simulink model "BESS_Harness"  (R2025b)
settings: Solver=VariableStepAuto  StartTime=0.0  StopTime=5  RelTol=1e-3
PostLoadFcn:
  | BESSParam
undefined symbols (not defined in the file): bessSystem, bessVoltage, DiscIntNeverNeededParam, gflInverter, gfmInverter, solar, Ts
libraries: eeGeneralControl x26, nesl_utility x26, ee_lib x16, simulink x12, fl_lib x10, eeTransforms x7, nesl_utility_internal x4, slpidlib x2, batteryecm_lib x2, simulink_extras x1, eePowerMeasurement x1, eePwmGenerator x1
(part 2 of 4)

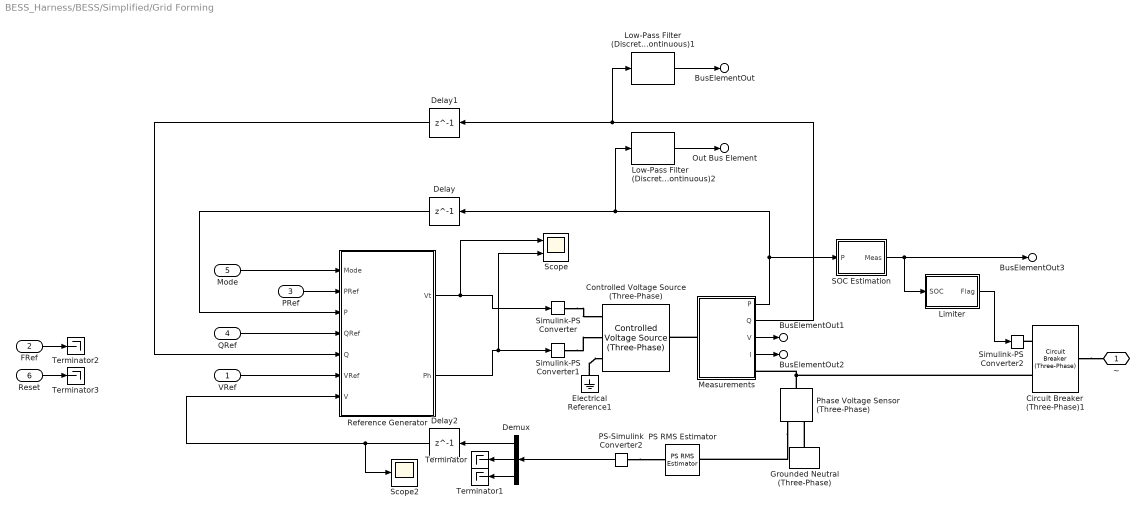
== system BESS_Harness/BESS/Simplified/Grid Forming ==
  VRef : Inport
  FRef : Inport  Port=2
  PRef : Inport  Port=3
  QRef : Inport  Port=4
  Mode : Inport  Port=5
  Reset : Inport  Port=6
  Circuit Breaker (Three-Phase)1 : ee_lib/Switches & Breakers/Circuit Breaker (Three-Phase)  R_closed=0.001 Ohm  G_open=1e-6 1/Ohm  threshold=0.5 V  breaker_behavior=ee.enum.switches.breakerBehavior.zeroCrossingDisable
      settings: InternalSimscapePortConfiguration="{\"Bottom\":[],\"Left\":[{\"id\":\"vT\",\"label\":\"vT\",\"type\":\"input\"},{\"id\":\"N1\",\"label\":\"~1\",\"type\":\"foundation.electrical.three_phase\"}],\"Right\":[{\"id\":\"N2\",\"label\":\"~2\",\"type\":\"foundation.electrical.three_phase\"}],\"Top\":[]}"
  Controlled Voltage Source (Three-Phase) : ee_lib/Sources/Controlled Voltage Source (Three-Phase)  input_option=ee.enum.inputType.singleFreqAC  FRated=frequency Hz
      settings: InternalSimscapePortConfiguration="{\"Bottom\":[],\"Left\":[{\"id\":\"Vt\",\"label\":\"Vt\",\"type\":\"input\"},{\"id\":\"ph\",\"label\":\"ph\",\"type\":\"input\"},{\"id\":\"n\",\"label\":\"n\",\"type\":\"foundation.electrical.electrical\"}],\"Right\":[{\"id\":\"N\",\"label\":\"~\",\"type\":\"foundation.electrical.three_phase\"}],\"Top\":[]}"
  Delay : Delay  DelayLength=1
  Delay1 : Delay  DelayLength=1
  Delay2 : Delay  DelayLength=1
  Demux : Demux  Outputs=3
  Electrical Reference1 : fl_lib/Electrical/Electrical Elements/Electrical Reference
  Grounded Neutral (Three-Phase) : ee_lib/Connectors & References/Grounded Neutral (Three-Phase)
  Limiter : Subsystem
  Low-Pass Filter (Discrete or Continuous)1 : eeGeneralControl/Low-Pass Filter (Discrete or Continuous)  K=1  T=0.1  B=inf  A=-inf  init_option=Inherited from block input  x0=0  Ts=-1
  Low-Pass Filter (Discrete or Continuous)2 : eeGeneralControl/Low-Pass Filter (Discrete or Continuous)  K=1  T=0.1  B=inf  A=-inf  init_option=Inherited from block input  x0=0  Ts=-1
  Measurements : Subsystem
  PS RMS Estimator : fl_lib/Physical Signals/Periodic Operators/PS RMS Estimator  f0=frequency Hz
      settings: InternalSimscapePortConfiguration="{\"Bottom\":[],\"Left\":[{\"id\":\"I\",\"label\":\"\",\"type\":\"input\"}],\"Right\":[{\"id\":\"O\",\"label\":\"\",\"type\":\"output\"}],\"Top\":[]}"
  PS-Simulink Converter2 : nesl_utility/PS-Simulink Converter  PhysicalDomain=network_engine_domain  SubClassName=ps_output  LeftPortType=input  RightPortType=output  PseudoPeriodic=off  Frequencies=[]  VectorFormat=inherit  Unit=inherit  AffineConversion=off
  Phase Voltage Sensor (Three-Phase) : ee_lib/Sensors & Transducers/Phase Voltage Sensor (Three-Phase)
  Reference Generator : Subsystem  mask{activeDroop=activeDroop, reactiveDroop=reactiveDroop, systemVoltage=Vac, systemFrequency=frequency, basePower=plantRating*1000}
      mask prompts: activeDroop "Active Droop"; reactiveDroop "Reactive Droop"; systemVoltage "AC Voltage"; systemFrequency "Frequency"; basePower "Base Power"
  SOC Estimation : Subsystem
  Scope : Scope  NumInputPorts=2
      settings: ActiveDisplayYMinimum=603.75  ActiveDisplayYMaximum=776.25000000000011
  Scope2 : Scope
  Simulink-PS Converter : nesl_utility/Simulink-PS Converter  PhysicalDomain=network_engine_domain  SubClassName=ps_input  LeftPortType=input  RightPortType=output  PseudoPeriodic=off  Frequencies=[]  NoiseDistribution=none  NoiseParameters=[]  Unit=1  AffineConversion=off  FilteringAndDerivatives=provide  SimscapeFilterOrder=1  InputFilterTimeConstant=0.001  UdotUserProvided=0
  Simulink-PS Converter1 : nesl_utility/Simulink-PS Converter  PhysicalDomain=network_engine_domain  SubClassName=ps_input  LeftPortType=input  RightPortType=output  PseudoPeriodic=off  Frequencies=[]  NoiseDistribution=none  NoiseParameters=[]  Unit=1  AffineConversion=off  FilteringAndDerivatives=provide  SimscapeFilterOrder=1  InputFilterTimeConstant=0.001  UdotUserProvided=0
  Simulink-PS Converter2 : nesl_utility/Simulink-PS Converter  PhysicalDomain=network_engine_domain  SubClassName=ps_input  LeftPortType=input  RightPortType=output  PseudoPeriodic=off  Frequencies=[]  NoiseDistribution=none  NoiseParameters=[]  Unit=1  AffineConversion=off  FilteringAndDerivatives=provide  SimscapeFilterOrder=1  InputFilterTimeConstant=0.001  UdotUserProvided=0
  Terminator{,1..3} (4 alike) : Terminator
  ~ : PMIOPort  Side=Right
  Out Bus Element : Outport  PortName=Meas  Element=activePower
  BusElementOut : Outport  PortName=Meas  Element=reactivePower
  BusElementOut1 : Outport  PortName=Meas  Element=voltage
  BusElementOut2 : Outport  PortName=Meas  Element=current
  BusElementOut3 : Outport  PortName=Meas  Element=SOC
  wires:
  Limiter/1(Flag) -> Simulink-PS Converter2/1
  PRef/1 -> Reference Generator/2(PRef)
  Low-Pass Filter (Discrete or Continuous)2/1 -> Out Bus Element/1
  Low-Pass Filter (Discrete or Continuous)1/1 -> BusElementOut/1
  Mode/1 -> Reference Generator/1(Mode)
  Delay1/1 -> Reference Generator/5(Q)
  FRef/1 -> Terminator2/1
  Reference Generator/1(Vt) -> Scope/1, Simulink-PS Converter/1
  VRef/1 -> Reference Generator/6(VRef)
  QRef/1 -> Reference Generator/4(QRef)
  Demux/1 -> Delay2/1
  Delay/1 -> Reference Generator/3(P)
  PS-Simulink Converter2/1 -> Demux/1
  Reference Generator/2(Ph) -> Scope/2, Simulink-PS Converter1/1
  Demux/2 -> Terminator/1
  Delay2/1 -> Reference Generator/7(V), Scope2/1
  Reset/1 -> Terminator3/1
  Demux/3 -> Terminator1/1
  Measurements/1(P) -> SOC Estimation/1(P), Low-Pass Filter (Discrete or Continuous)2/1, Delay/1
  Measurements/2(Q) -> Low-Pass Filter (Discrete or Continuous)1/1, Delay1/1
  Measurements/3(V) -> BusElementOut1/1
  Measurements/4(I) -> BusElementOut2/1
  SOC Estimation/1(Meas) -> Limiter/1(SOC), BusElementOut3/1
  connections:
  Circuit Breaker (Three-Phase)1/LConn1 -- Simulink-PS Converter2/RConn1
  Circuit Breaker (Three-Phase)1/RConn1 -- ~/RConn1
  PS-Simulink Converter2/LConn1 -- PS RMS Estimator/RConn1
  Measurements/LConn1 -- Controlled Voltage Source (Three-Phase)/RConn1
  Simulink-PS Converter1/RConn1 -- Controlled Voltage Source (Three-Phase)/LConn2
  Electrical Reference1/LConn1 -- Controlled Voltage Source (Three-Phase)/LConn3
  Circuit Breaker (Three-Phase)1/LConn2 -- Phase Voltage Sensor (Three-Phase)/LConn1 -- Measurements/RConn1
  Phase Voltage Sensor (Three-Phase)/RConn1 -- PS RMS Estimator/LConn1
  Simulink-PS Converter/RConn1 -- Controlled Voltage Source (Three-Phase)/LConn1
  Grounded Neutral (Three-Phase)/LConn1 -- Phase Voltage Sensor (Three-Phase)/RConn2

== system BESS_Harness/BESS/Detailed/BESS Controller/Grid Following ==
  VRef : Inport
  FRef : Inport  Port=2
  PRef : Inport  Port=3
  QRef : Inport  Port=4
  Mode : Inport  Port=5
  Reset : Inport  Port=6
  In Bus Element3 : Inport  Port=7  PortName=VIBus  Element=Vd
  BusElementIn : Inport  Port=7  PortName=VIBus  Element=Vd
  In Bus Element2 : Inport  Port=7  PortName=VIBus  Element=Vq
  In Bus Element7 : Inport  Port=7  PortName=VIBus  Element=Theta
  BusElementIn1 : Inport  Port=7  PortName=VIBus  Element=Freq
  BusElementIn3 : Inport  Port=7  PortName=VIBus  Element=Id
  BusElementIn4 : Inport  Port=7  PortName=VIBus  Element=Iq
  Constant : Constant  Value=10
  Current_controller : Subsystem
  Inverse Park Transform1 : eeTransforms/Inverse Park Transform  AxisAlignment=Q-axis  PowerInvariant=off
  Reference Current : Subsystem
  Sum2 : Sum  Inputs=|+-
  Terminator : Terminator
  Terminator1 : Terminator
  Unit Delay : UnitDelay  SampleTime=Td
  Unit Delay1 : UnitDelay  SampleTime=Td
  Unit Delay2 : UnitDelay  SampleTime=Ts
  mabc : Outport
  wires:
  QRef/1 -> Reference Current/6(QRef)
  PRef/1 -> Reference Current/5(PRef)
  BusElementIn4/1 -> Current_controller/4(iq)
  BusElementIn3/1 -> Current_controller/2(ipvd)
  BusElementIn1/1 -> Unit Delay1/1
  BusElementIn/1 -> Unit Delay/1
  Unit Delay/1 -> Reference Current/2(V-mag)
  Unit Delay1/1 -> Sum2/2
  Reference Current/1(id_ref) -> Current_controller/1(id-ref)
  Reference Current/2(iq_ref) -> Current_controller/3(iqref)
  Sum2/1 -> Reference Current/3(del f)
  VRef/1 -> Reference Current/1(V_ref)
  FRef/1 -> Sum2/1
  In Bus Element7/1 -> Inverse Park Transform1/2
  In Bus Element3/1 -> Current_controller/5(Vd)
  Current_controller/1(mdq0) -> Inverse Park Transform1/1
  Unit Delay2/1 -> mabc/1
  Inverse Park Transform1/1 -> Unit Delay2/1
  In Bus Element2/1 -> Current_controller/6(Vq)
  Mode/1 -> Terminator/1
  Reset/1 -> Terminator1/1
  Constant/1 -> Reference Current/4(LVRT_iq)

== system BESS_Harness/BESS/Detailed/BESS Controller/Grid Forming ==
  VRef : Inport
  FRef : Inport  Port=2
  PRef : Inport  Port=3
  QRef : Inport  Port=4
  Mode : Inport  Port=5
  Reset : Inport  Port=6
  Bus Element In : Inport  Port=7  PortName=VIBus  Element=Vabc
  BusElementIn : Inport  Port=7  PortName=VIBus  Element=Iabc
  Current Limiting : Subsystem
  Grid Voltage Reactive Power Support : Subsystem
  Measurement : Subsystem
      mask Display: image('meas2_1_7_7_2.png');
  Power Control : Subsystem
  Subsystem2 : Subsystem
      settings: PortSchema="{\"entries\":[{\"content\":{\"sides\":[{\"content\":{\"connectorIds\":[\"Out1\"]},\"type\":\"ConnectorPlacement.EquallySpacedRectSide\",\"uuid\":\"7526c1f7-0aba-4355-8bbd-47d168879ecb\"},{\"content\":{\"connectorIds\":[\"In1\",\"In2\"],\"side\":\"RIGHT\"},\"type\":\"ConnectorPlacement.EquallySpacedRectSide\",\"uuid\":\"1dda9693-ec76-4df0-8ad4-aaa83d2574b3\"},{\"content\":{\"side\":\"TOP\"},\"type\":\"ConnectorPlacement.EquallySpacedRectSide\",\"uuid\":\"71ea411b-eb5f-4279-ae23-08ebb3ff1ed6\"}]},\"type\":\"ConnectorPlacement.EquallySpacedConnector\",\"uuid\":\"19864e0c-0998-460d-9705-13c69283d4ec\"}],\"packageUris\":[\"http://schema.mathworks.com/mf0/Connector/R2020b\"],\"version\":\"1.0\"}"
  Terminator : Terminator
  Terminator1 : Terminator
  Terminator2 : Terminator
  VoltageCurrentControl : Subsystem
      settings: PortSchema="{\"entries\":[{\"content\":{\"sides\":[{\"content\":{\"connectorIds\":[\"In1\",\"In2\",\"In3\"]},\"type\":\"ConnectorPlacement.EquallySpacedRectSide\",\"uuid\":\"0bf15a12-7bc0-47e4-89bd-435769673763\"},{\"content\":{\"connectorIds\":[\"Out1\"],\"side\":\"RIGHT\"},\"type\":\"ConnectorPlacement.EquallySpacedRectSide\",\"uuid\":\"44a15d74-8878-4ec6-abe4-be0b1b609519\"},{\"content\":{\"connectorIds\":[\"In4\"],\"side\":\"TOP\"},\"type\":\"ConnectorPlacement.EquallySpacedRectSide\",\"uuid\":\"7a96781e-5638-4b2a-8101-d5785aae9f0f\"}]},\"type\":\"ConnectorPlacement.EquallySpacedConnector\",\"uuid\":\"4b3373ad-cf20-4175-894e-3bd1604dd0ce\"}],\"packageUris\":[\"http://schema.mathworks.com/mf0/Connector/R2020b\"],\"version\":\"1.0\"}"
  mabc : Outport
  wires:
  Reset/1 -> Subsystem2/2(Reset), VoltageCurrentControl/3(Reset)
  Mode/1 -> Power Control/6(CntrlFlag)
  VRef/1 -> Power Control/4(Vref)
  FRef/1 -> Power Control/5(Fref)
  Measurement/4(fmeas) -> Terminator2/1
  Grid Voltage Reactive Power Support/2(Qref) -> Power Control/3(Qref)
  Grid Voltage Reactive Power Support/1(Pref) -> Power Control/2(Pref)
  PRef/1 -> Grid Voltage Reactive Power Support/2(PrefInput)
  QRef/1 -> Grid Voltage Reactive Power Support/3(QrefInput)
  Current Limiting/1(currentLimiting) -> VoltageCurrentControl/1(currentLimiting)
  Power Control/2(activeControl) -> VoltageCurrentControl/2(activeControl)
  Power Control/1(reactiveControl) -> Current Limiting/2(reactiveControl)
  Power Control/3(angle) -> Measurement/3(Angle)
  Measurement/1(measure) -> Grid Voltage Reactive Power Support/1(measure), Power Control/1(measure), VoltageCurrentControl/4(measure), Current Limiting/1(measure)
  Measurement/3(Qmeas) -> Terminator1/1
  Measurement/2(Pmeas) -> Terminator/1
  BusElementIn/1 -> Measurement/2(Igabc)
  Bus Element In/1 -> Measurement/1(Vgabcc)
  VoltageCurrentControl/1(mabc) -> Subsystem2/1(In)
  Subsystem2/1(mabc) -> mabc/1

== system BESS_Harness/BESS/Detailed/BESS Plant/Converter ==
  mabc : Inport
  Average : Subsystem  VariantControl=Average
  Switching : Subsystem  VariantControl=Switching
  + : PMIOPort  Side=Left
  - : PMIOPort  Port=2  Side=Left
  ~ : PMIOPort  Port=3  Side=Right

== system BESS_Harness/BESS/Detailed/Filter & Measurements/PLL & Measurements ==
  V : Inport
  I : Inport  Port=2
  Measurement1 : Subsystem
  Measurement2 : Subsystem
  Subsystem : Subsystem
  Out Bus Element : Outport  PortName=VIbus  Element=Vq
  Out Bus Element1 : Outport  PortName=VIbus  Element=Vd
  Out Bus Element2 : Outport  PortName=VIbus  Element=Freq
  Out Bus Element3 : Outport  PortName=VIbus  Element=Theta
  Out Bus Element4 : Outport  PortName=VIbus  Element=Vmag
  Out Bus Element5 : Outport  PortName=VIbus  Element=Iq
  Out Bus Element6 : Outport  PortName=VIbus  Element=Id
  Out Bus Element7 : Outport  PortName=VIbus  Element=Iabc
  Out Bus Element8 : Outport  PortName=VIbus  Element=Vabc
  wires:
  Subsystem/6(Id1) -> Out Bus Element6/1
  Subsystem/7(Iq1) -> Out Bus Element5/1
  Measurement1/1(Vg) -> Subsystem/2(Iabc), Out Bus Element7/1
  I/1 -> Measurement1/1(u)
  Subsystem/1(mag) -> Out Bus Element4/1
  Measurement2/1(Vg) -> Subsystem/1(Vabc), Out Bus Element8/1
  Subsystem/4(Vd) -> Out Bus Element1/1
  Subsystem/3(angle) -> Out Bus Element3/1
  Subsystem/5(Vq) -> Out Bus Element/1
  Subsystem/2(freq) -> Out Bus Element2/1
  V/1 -> Measurement2/1(u)

== system BESS_Harness/BESS/Simplified/Grid Following/Measurements ==
  Current and Voltage Sensor (Three-Phase)1 : ee_lib/Sensors & Transducers/Current and Voltage Sensor (Three-Phase)  vMeasurementType=ee.enum.vmeasurement.lg  outputUnit=ee.enum.unit.pu  SRated=plantRating*1000 A*V  VRated=Vac V  I_specify=off  I_priority=None  I=[0, 0, 0] A  I_nominal_specify=off  I_nominal_value=1  I_nominal_unit=A  V_specify=off  V_priority=None  V=[0, 0, 0] V  V_nominal_specify=off  V_nominal_value=1  V_nominal_unit=V
      settings: InternalSimscapePortConfiguration="{\"Bottom\":[],\"Left\":[{\"id\":\"N1\",\"label\":\"~1\",\"type\":\"foundation.electrical.three_phase\"}],\"Right\":[{\"id\":\"V_output\",\"label\":\"V\",\"type\":\"output\"},{\"id\":\"I_output\",\"label\":\"I\",\"type\":\"output\"},{\"id\":\"N2\",\"label\":\"~2\",\"type\":\"foundation.electrical.three_phase\"}],\"Top\":[]}"
  Gain1 : Gain  Gain=1/(plantRating*1000)
  Gain2 : Gain  Gain=1/(plantRating*1000)
  Low-Pass Filter (Discrete or Continuous)1 : eeGeneralControl/Low-Pass Filter (Discrete or Continuous)  K=1  T=0.1  B=inf  A=-inf  init_option=Inherited from block input  x0=0  Ts=-1
  Low-Pass Filter (Discrete or Continuous)2 : eeGeneralControl/Low-Pass Filter (Discrete or Continuous)  K=1  T=0.1  B=inf  A=-inf  init_option=Inherited from block input  x0=0  Ts=-1
  PS-Simulink Converter{,1..3} (4 alike) : nesl_utility/PS-Simulink Converter  PhysicalDomain=network_engine_domain  SubClassName=ps_output  LeftPortType=input  RightPortType=output  PseudoPeriodic=off  Frequencies=[]  VectorFormat=inherit  Unit=inherit  AffineConversion=off
  Power Sensor (Three-Phase) : ee_lib/Sensors & Transducers/Power Sensor (Three-Phase)  load_type=ee.enum.passive.type_balanced.balanced  f0=60 Hz
      settings: InternalSimscapePortConfiguration="{\"Bottom\":[],\"Left\":[{\"id\":\"N1\",\"label\":\"~1\",\"type\":\"foundation.electrical.three_phase\"}],\"Right\":[{\"id\":\"N2\",\"label\":\"~2\",\"type\":\"foundation.electrical.three_phase\"}],\"Top\":[{\"id\":\"Pm\",\"label\":\"P\",\"type\":\"output\"},{\"id\":\"Qm\",\"label\":\"Q\",\"type\":\"output\"}]}"
  In : PMIOPort  Side=Left
  ~ : PMIOPort  Port=2  Side=Right
  P : Outport
  Q : Outport  Port=2
  V : Outport  Port=3
  I : Outport  Port=4
  wires:
  Gain2/1 -> Q/1
  Gain1/1 -> P/1
  PS-Simulink Converter3/1 -> I/1
  PS-Simulink Converter2/1 -> V/1
  Low-Pass Filter (Discrete or Continuous)2/1 -> Gain2/1
  Low-Pass Filter (Discrete or Continuous)1/1 -> Gain1/1
  PS-Simulink Converter1/1 -> Low-Pass Filter (Discrete or Continuous)2/1
  PS-Simulink Converter/1 -> Low-Pass Filter (Discrete or Continuous)1/1
  connections:
  Current and Voltage Sensor (Three-Phase)1/RConn2 -- PS-Simulink Converter3/LConn1
  Current and Voltage Sensor (Three-Phase)1/LConn1 -- Power Sensor (Three-Phase)/RConn1
  PS-Simulink Converter1/LConn1 -- Power Sensor (Three-Phase)/LConn3
  Current and Voltage Sensor (Three-Phase)1/RConn3 -- ~/RConn1
  In/RConn1 -- Power Sensor (Three-Phase)/LConn1
  PS-Simulink Converter/LConn1 -- Power Sensor (Three-Phase)/LConn2
  Current and Voltage Sensor (Three-Phase)1/RConn1 -- PS-Simulink Converter2/LConn1

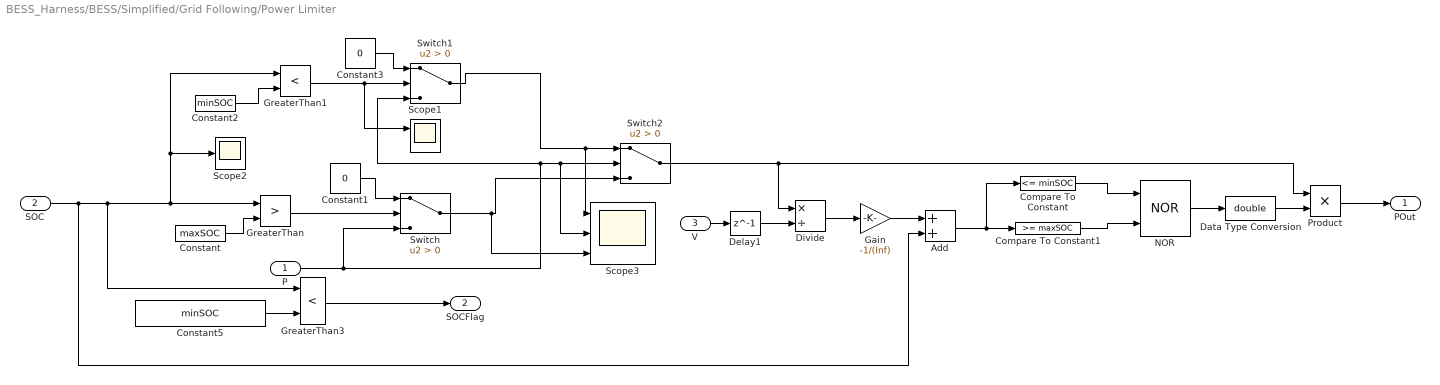
== system BESS_Harness/BESS/Simplified/Grid Following/Power Limiter ==
  P : Inport
  SOC : Inport  Port=2
  V : Inport  Port=3
  Add : Sum
  Compare To Constant : simulink/Logic and Bit Operations/Compare To Constant  relop=<=  const=minSOC  OutDataTypeStr=boolean
  Compare To Constant1 : simulink/Logic and Bit Operations/Compare To Constant  relop=>=  const=maxSOC  OutDataTypeStr=boolean
  Constant : Constant  Value=maxSOC
  Constant1 : Constant  Value=0
  Constant2 : Constant  Value=minSOC
  Constant3 : Constant  Value=0
  Constant5 : Constant  Value=minSOC
  Data Type Conversion : DataTypeConversion  OutDataTypeStr=double  SaturateOnIntegerOverflow=off  RndMeth=Floor
  Delay1 : Delay  DelayLength=1
  Divide : Product  Inputs=*/
  Gain : Gain  Gain=-1/(Inf)
  GreaterThan : RelationalOperator  Operator=>  OutDataTypeStr=boolean  RndMeth=Simplest  InputSameDT=off
  GreaterThan1 : RelationalOperator  Operator=<  OutDataTypeStr=boolean  RndMeth=Simplest  InputSameDT=off
  GreaterThan3 : RelationalOperator  Operator=<  OutDataTypeStr=boolean  RndMeth=Simplest  InputSameDT=off
  NOR : Logic  Operator=NOR  IconShape=distinctive  AllPortsSameDT=off  OutDataTypeStr=boolean
  Product : Product
  Scope1 : Scope  NumInputPorts=2
  Scope2 : Scope
  Scope3 : Scope  NumInputPorts=3
  Switch : Switch  Criteria=u2 > Threshold  SaturateOnIntegerOverflow=off  InputSameDT=off
  Switch1 : Switch  Criteria=u2 > Threshold  SaturateOnIntegerOverflow=off  InputSameDT=off
  Switch2 : Switch  Criteria=u2 > Threshold  SaturateOnIntegerOverflow=off  InputSameDT=off
  POut : Outport
  SOCFlag : Outport  Port=2
  wires:
  Product/1 -> POut/1
  Gain/1 -> Add/1
  Data Type Conversion/1 -> Product/2
  NOR/1 -> Data Type Conversion/1
  Compare To Constant1/1 -> NOR/2
  Compare To Constant/1 -> NOR/1
  Add/1 -> Compare To Constant1/1, Compare To Constant/1
  Switch2/1 -> Product/1, Divide/1
  Switch/1 -> Switch2/3, Scope3/3
  SOC/1 -> GreaterThan/1, GreaterThan1/1, Scope2/1, GreaterThan3/1, Add/2
  Divide/1 -> Gain/1
  Delay1/1 -> Divide/2
  V/1 -> Delay1/1
  GreaterThan3/1 -> SOCFlag/1
  Constant5/1 -> GreaterThan3/2
  Constant/1 -> GreaterThan/2
  GreaterThan/1 -> Switch/2
  Constant1/1 -> Switch/1
  Constant2/1 -> GreaterThan1/2
  GreaterThan1/1 -> Switch1/2, Scope1/1
  Constant3/1 -> Switch1/1
  Switch1/1 -> Switch2/1, Scope3/1
  P/1 -> Switch/3, Switch1/3, Switch2/2, Scope3/2

== system BESS_Harness/BESS/Simplified/Grid Following/SOC Estimation ==
  I : Inport
  Constant : Constant  Value=0.95
  Gain : Gain  Gain=-1/(100000)
  Integrator (Discrete or Continuous) : eeGeneralControl/Integrator (Discrete or Continuous)  LabelModeActiveChoice=Discrete  IntegratorMethod=Integration: Forward Euler  ExternalReset=level  LimitType=Anti-windup  B=inf  A=-inf  Ts=-1
  SOC : Outport
  wires:
  Integrator (Discrete or Continuous)/1 -> SOC/1
  Gain/1 -> Integrator (Discrete or Continuous)/1
  I/1 -> Gain/1
  Constant/1 -> Integrator (Discrete or Continuous)/3

== system BESS_Harness/BESS/Simplified/Grid Forming/Limiter ==
  SOC : Inport
  Compare To Constant : simulink/Logic and Bit Operations/Compare To Constant  relop=<=  const=minSOC  OutDataTypeStr=boolean
  Compare To Constant1 : simulink/Logic and Bit Operations/Compare To Constant  relop=>=  const=maxSOC  OutDataTypeStr=boolean
  Data Type Conversion : DataTypeConversion  OutDataTypeStr=double  SaturateOnIntegerOverflow=off  RndMeth=Floor
  Delay : Delay  DelayLength=1  InputProcessing=Columns as channels (frame based)
  OR : Logic  Operator=OR  AllPortsSameDT=off  OutDataTypeStr=boolean
  Flag : Outport
  wires:
  Delay/1 -> Flag/1
  Data Type Conversion/1 -> Delay/1
  OR/1 -> Data Type Conversion/1
  Compare To Constant1/1 -> OR/2
  Compare To Constant/1 -> OR/1
  SOC/1 -> Compare To Constant1/1, Compare To Constant/1

== system BESS_Harness/BESS/Simplified/Grid Forming/Measurements ==
  Current and Voltage Sensor (Three-Phase)5 : ee_lib/Sensors & Transducers/Current and Voltage Sensor (Three-Phase)  vMeasurementType=ee.enum.vmeasurement.lg  outputUnit=ee.enum.unit.pu  SRated=plantRating*1000 A*V  VRated=Vac V  I_specify=off  I_priority=None  I=[0, 0, 0] A  I_nominal_specify=off  I_nominal_value=1  I_nominal_unit=A  V_specify=off  V_priority=None  V=[0, 0, 0] V  V_nominal_specify=off  V_nominal_value=1  V_nominal_unit=V
      settings: InternalSimscapePortConfiguration="{\"Bottom\":[],\"Left\":[{\"id\":\"N1\",\"label\":\"~1\",\"type\":\"foundation.electrical.three_phase\"}],\"Right\":[{\"id\":\"V_output\",\"label\":\"V\",\"type\":\"output\"},{\"id\":\"I_output\",\"label\":\"I\",\"type\":\"output\"},{\"id\":\"N2\",\"label\":\"~2\",\"type\":\"foundation.electrical.three_phase\"}],\"Top\":[]}"
  Gain1 : Gain  Gain=1/(plantRating*1000)
  Gain2 : Gain  Gain=1/(plantRating*1000)
  PS-Simulink Converter{,1..3} (4 alike) : nesl_utility/PS-Simulink Converter  PhysicalDomain=network_engine_domain  SubClassName=ps_output  LeftPortType=input  RightPortType=output  PseudoPeriodic=off  Frequencies=[]  VectorFormat=inherit  Unit=inherit  AffineConversion=off
  Power Sensor (Three-Phase) : ee_lib/Sensors & Transducers/Power Sensor (Three-Phase)  load_type=ee.enum.passive.type_balanced.balanced  f0=60 Hz
      settings: InternalSimscapePortConfiguration="{\"Bottom\":[],\"Left\":[{\"id\":\"N1\",\"label\":\"~1\",\"type\":\"foundation.electrical.three_phase\"}],\"Right\":[{\"id\":\"N2\",\"label\":\"~2\",\"type\":\"foundation.electrical.three_phase\"}],\"Top\":[{\"id\":\"Pm\",\"label\":\"P\",\"type\":\"output\"},{\"id\":\"Qm\",\"label\":\"Q\",\"type\":\"output\"}]}"
  In : PMIOPort  Side=Left
  ~ : PMIOPort  Port=2  Side=Right
  P : Outport
  Q : Outport  Port=2
  V : Outport  Port=3
  I : Outport  Port=4
  wires:
  PS-Simulink Converter1/1 -> Gain2/1
  PS-Simulink Converter/1 -> Gain1/1
  PS-Simulink Converter2/1 -> V/1
  PS-Simulink Converter3/1 -> I/1
  Gain1/1 -> P/1
  Gain2/1 -> Q/1
  connections:
  PS-Simulink Converter2/LConn1 -- Current and Voltage Sensor (Three-Phase)5/RConn1
  PS-Simulink Converter/LConn1 -- Power Sensor (Three-Phase)/LConn2
  In/RConn1 -- Power Sensor (Three-Phase)/LConn1
  ~/RConn1 -- Current and Voltage Sensor (Three-Phase)5/RConn3
  PS-Simulink Converter1/LConn1 -- Power Sensor (Three-Phase)/LConn3
  Power Sensor (Three-Phase)/RConn1 -- Current and Voltage Sensor (Three-Phase)5/LConn1
  PS-Simulink Converter3/LConn1 -- Current and Voltage Sensor (Three-Phase)5/RConn2

== system BESS_Harness/BESS/Simplified/Grid Forming/Reference Generator ==
  Mode : Inport
  PRef : Inport  Port=2
  P : Inport  Port=3
  QRef : Inport  Port=4
  Q : Inport  Port=5
  VRef : Inport  Port=6
  V : Inport  Port=7
  Gain : Gain  Gain=efficiency/100
  Gain2 : Gain  Gain=sqrt(3)/Vac
  If : If
  If Action Subsystem : Subsystem  TreatAsAtomicUnit=on
  If Action Subsystem1 : Subsystem  TreatAsAtomicUnit=on
  Merge : Merge
  Merge1 : Merge
  Vt : Outport
  Ph : Outport  Port=2
  wires:
  Gain/1 -> If Action Subsystem/1(PRef)
  Mode/1 -> If/1
  If/1 -> If Action Subsystem/Action
  PRef/1 -> Gain/1, If Action Subsystem1/1(PRef)
  QRef/1 -> If Action Subsystem/3(QRef)
  VRef/1 -> If Action Subsystem1/3(VRef)
  V/1 -> Gain2/1
  If/2 -> If Action Subsystem1/Action
  If Action Subsystem/1(Vt) -> Merge/1
  If Action Subsystem1/1(Vt) -> Merge/2
  If Action Subsystem/2(Ph) -> Merge1/1
  If Action Subsystem1/2(Ph) -> Merge1/2
  Merge1/1 -> Ph/1
  P/1 -> If Action Subsystem/2(P), If Action Subsystem1/2(P)
  Q/1 -> If Action Subsystem/4(Q)
  Gain2/1 -> If Action Subsystem1/4(V)
  Merge/1 -> Vt/1

== system BESS_Harness/BESS/Simplified/Grid Forming/SOC Estimation ==
  P : Inport
  Constant : Constant  Value=Vdc
  Constant1 : Constant  Value=initialSOC
  Constant2 : Constant  Value=capacity
  Constant3 : Constant  Value=Inf
  Divide : Product  Inputs=*/
  Divide1 : Product  Inputs=*/
  Gain : Gain  Gain=-plantRating*1000
  Integrator (Discrete or Continuous) : eeGeneralControl/Integrator (Discrete or Continuous)  LabelModeActiveChoice=Discrete  IntegratorMethod=Integration: Forward Euler  ExternalReset=level  LimitType=Anti-windup  B=inf  A=-inf  Ts=-1
  String Compare : StringCompare
  String Constant : StringConstant  String=capacityType
  String Constant1 : StringConstant  String="\"Fixed\""
  Switch : Switch  Criteria=u2 > Threshold  SaturateOnIntegerOverflow=off  InputSameDT=off
  Meas : Outport
  wires:
  Gain/1 -> Divide/1
  P/1 -> Gain/1
  Constant/1 -> Divide/2
  Divide/1 -> Divide1/1
  Constant1/1 -> Integrator (Discrete or Continuous)/3
  Integrator (Discrete or Continuous)/1 -> Meas/1
  String Constant/1 -> String Compare/1
  String Constant1/1 -> String Compare/2
  String Compare/1 -> Switch/2
  Switch/1 -> Divide1/2
  Divide1/1 -> Integrator (Discrete or Continuous)/1
  Constant2/1 -> Switch/1
  Constant3/1 -> Switch/3

== system BESS_Harness/BESS/Detailed/BESS Controller/Grid Following/Current_controller ==
  id-ref : Inport
  ipvd : Inport  Port=2
  iqref : Inport  Port=3
  iq : Inport  Port=4
  Vd : Inport  Port=5
  Vq : Inport  Port=6
  Constant4 : Constant  Value=0
  Gain1 : Gain  Gain=2*1*pi*frequency*L/zbase
  Gain2 : Gain  Gain=2*1*pi*frequency*L/zbase
  Mux1 : Mux  Inputs=3
  PID Controller : slpidlib/PID Controller  Controller=PID  Form=Parallel  TimeDomain=Discrete-time  UseExternalTs=off  SampleTime=-1  IntegratorMethod=Forward Euler  FilterMethod=Forward Euler  ControllerParametersSource=internal  P=Kpic  I=Kiic  UseKiTs=off  D=Kd  UseExternalDerivativeSource=off  N=100  UseFilter=on  TunerSelectOption=Transfer Function Based (PID Tuner App)  InitialConditionSource=internal  InitialConditionForIntegrator=0  InitialConditionForFilter=0  DifferentiatorICPrevScaledInput=0  ExternalReset=none  TrackingMode=off  Kt=1  LimitOutput=off  SatLimitsSource=internal  UpperSaturationLimit=inf  LowerSaturationLimit=-inf  LinearizeAsGain=on  AntiWindupMode=none  Kb=1  LimitIntegrator=off  UpperIntegratorSaturationLimit=inf  LowerIntegratorSaturationLimit=-inf  POutMin=[]  POutMax=[]  IOutMin=[]  IOutMax=[]  DOutMin=[]  DOutMax=[]  NOutMin=[]  NOutMax=[]  SumOutMin=[]  SumOutMax=[]  SaturationOutMin=[]  SaturationOutMax=[]  PParamMin=[]  PParamMax=[]  IParamMin=[]  IParamMax=[]  DParamMin=[]  DParamMax=[]  NParamMin=[]  NParamMax=[]  KbParamMin=[]  KbParamMax=[]  KtParamMin=[]  KtParamMax=[]  KbOutMin=[]  KbOutMax=[]  KtOutMin=[]  KtOutMax=[]  IntegratorOutMin=[]  IntegratorOutMax=[]  FilterOutMin=[]  FilterOutMax=[]  SumI1OutMin=[]  SumI1OutMax=[]  SumI2OutMin=[]  SumI2OutMax=[]  SumI3OutMin=[]  SumI3OutMax=[]  SumI4OutMin=[]  SumI4OutMax=[]  SumDOutMin=[]  SumDOutMax=[]  DifferentiatorOutMin=[]  DifferentiatorOutMax=[]  FilterDiffOutCoefMin=[]  FilterDiffOutCoefMax=[]  ReciprocalOutMin=[]  ReciprocalOutMax=[]  SumDenOutMin=[]  SumDenOutMax=[]  SumNumOutMin=[]  SumNumOutMax=[]  DivideOutMin=[]  DivideOutMax=[]  UdiffTsProdOutMin=[]  UdiffTsProdOutMax=[]  NTsProdOutMin=[]  NTsProdOutMax=[]  UintegralTsProdOutMin=[]  UintegralTsProdOutMax=[]  UngainTsProdOutMin=[]  UngainTsProdOutMax=[]  ClampingZeroOutDataTypeStr=Inherit: Inherit via back propagation  ClampingZeroOutMin=[]  ClampingZeroOutMax=[]  FilterDenConstantOutDataTypeStr=Inherit: Inherit via back propagation  FilterDenConstantOutMin=[]  FilterDenConstantOutMax=[]  PCopyOutDataTypeStr=Inherit: Inherit via back propagation  PCopyOutMin=[]  PCopyOutMax=[]  NCopyOutDataTypeStr=Inherit: Inherit via back propagation  NCopyOutMin=[]  NCopyOutMax=[]  IntegratorContinuousStateAttributes=''  IntegratorStateMustResolveToSignalObject=off  IntegratorRTWStateStorageClass=Auto  FilterContinuousStateAttributes=''  FilterStateMustResolveToSignalObject=off  FilterRTWStateStorageClass=Auto  ParallelPVariant=InternalParameters  IdealPVariant=Disabled  IVariant=InternalParameters  DVariant=InternalParameters  IntegratorVariant=Discrete  SatVariant=Disabled  AWVariant=Passthrough  PCopyVariant=Disabled  TRVariant=Disabled  FdbkBlocksVariant=Forward  IdealPFdbkVariant=Disabled  SatFdbkVariant=Disabled  DerivativeFilterVariant=ForwardEulerFilter  NVariant=InternalParameters  NCopyVariant=Disabled  FilterICVariant=InternalICsFilter  IntegratorICVariant=InternalICs  ExternalResetVariant=Disabled  TRSumVariant=Passthrough  SumFdbkVariant=Disabled  SumVariant=Sum_PID  TsampFilterVariant=InternalTs  TsampNgainVariant=Passthrough  TsampIntegralVariant=Disabled_SignalSpec  ExternalSaturationOutDataTypeStr=Inherit: Same as second input  DerivativeSourceVariant=ErrorSignal  PreIntVariant=InternalPreInt
  PID Controller1 : slpidlib/PID Controller  Controller=PID  Form=Parallel  TimeDomain=Discrete-time  UseExternalTs=off  SampleTime=-1  IntegratorMethod=Forward Euler  FilterMethod=Forward Euler  ControllerParametersSource=internal  P=Kpic  I=Kiic  UseKiTs=off  D=Kd  UseExternalDerivativeSource=off  N=100  UseFilter=on  TunerSelectOption=Transfer Function Based (PID Tuner App)  InitialConditionSource=internal  InitialConditionForIntegrator=0  InitialConditionForFilter=0  DifferentiatorICPrevScaledInput=0  ExternalReset=none  TrackingMode=off  Kt=1  LimitOutput=off  SatLimitsSource=internal  UpperSaturationLimit=inf  LowerSaturationLimit=-inf  LinearizeAsGain=on  AntiWindupMode=none  Kb=1  LimitIntegrator=off  UpperIntegratorSaturationLimit=inf  LowerIntegratorSaturationLimit=-inf  POutMin=[]  POutMax=[]  IOutMin=[]  IOutMax=[]  DOutMin=[]  DOutMax=[]  NOutMin=[]  NOutMax=[]  SumOutMin=[]  SumOutMax=[]  SaturationOutMin=[]  SaturationOutMax=[]  PParamMin=[]  PParamMax=[]  IParamMin=[]  IParamMax=[]  DParamMin=[]  DParamMax=[]  NParamMin=[]  NParamMax=[]  KbParamMin=[]  KbParamMax=[]  KtParamMin=[]  KtParamMax=[]  KbOutMin=[]  KbOutMax=[]  KtOutMin=[]  KtOutMax=[]  IntegratorOutMin=[]  IntegratorOutMax=[]  FilterOutMin=[]  FilterOutMax=[]  SumI1OutMin=[]  SumI1OutMax=[]  SumI2OutMin=[]  SumI2OutMax=[]  SumI3OutMin=[]  SumI3OutMax=[]  SumI4OutMin=[]  SumI4OutMax=[]  SumDOutMin=[]  SumDOutMax=[]  DifferentiatorOutMin=[]  DifferentiatorOutMax=[]  FilterDiffOutCoefMin=[]  FilterDiffOutCoefMax=[]  ReciprocalOutMin=[]  ReciprocalOutMax=[]  SumDenOutMin=[]  SumDenOutMax=[]  SumNumOutMin=[]  SumNumOutMax=[]  DivideOutMin=[]  DivideOutMax=[]  UdiffTsProdOutMin=[]  UdiffTsProdOutMax=[]  NTsProdOutMin=[]  NTsProdOutMax=[]  UintegralTsProdOutMin=[]  UintegralTsProdOutMax=[]  UngainTsProdOutMin=[]  UngainTsProdOutMax=[]  ClampingZeroOutDataTypeStr=Inherit: Inherit via back propagation  ClampingZeroOutMin=[]  ClampingZeroOutMax=[]  FilterDenConstantOutDataTypeStr=Inherit: Inherit via back propagation  FilterDenConstantOutMin=[]  FilterDenConstantOutMax=[]  PCopyOutDataTypeStr=Inherit: Inherit via back propagation  PCopyOutMin=[]  PCopyOutMax=[]  NCopyOutDataTypeStr=Inherit: Inherit via back propagation  NCopyOutMin=[]  NCopyOutMax=[]  IntegratorContinuousStateAttributes=''  IntegratorStateMustResolveToSignalObject=off  IntegratorRTWStateStorageClass=Auto  FilterContinuousStateAttributes=''  FilterStateMustResolveToSignalObject=off  FilterRTWStateStorageClass=Auto  ParallelPVariant=InternalParameters  IdealPVariant=Disabled  IVariant=InternalParameters  DVariant=InternalParameters  IntegratorVariant=Discrete  SatVariant=Disabled  AWVariant=Passthrough  PCopyVariant=Disabled  TRVariant=Disabled  FdbkBlocksVariant=Forward  IdealPFdbkVariant=Disabled  SatFdbkVariant=Disabled  DerivativeFilterVariant=ForwardEulerFilter  NVariant=InternalParameters  NCopyVariant=Disabled  FilterICVariant=InternalICsFilter  IntegratorICVariant=InternalICs  ExternalResetVariant=Disabled  TRSumVariant=Passthrough  SumFdbkVariant=Disabled  SumVariant=Sum_PID  TsampFilterVariant=InternalTs  TsampNgainVariant=Passthrough  TsampIntegralVariant=Disabled_SignalSpec  ExternalSaturationOutDataTypeStr=Inherit: Same as second input  DerivativeSourceVariant=ErrorSignal  PreIntVariant=InternalPreInt
  Scope : Scope  NumInputPorts=2
      settings: ActiveDisplayYMinimum=-1  ActiveDisplayYMaximum=1
  Scope1 : Scope  NumInputPorts=2
      settings: ActiveDisplayYMinimum=-1.21282  ActiveDisplayYMaximum=0.9154  DataLoggingVariableName=ScopeData2
  Sum1 : Sum  Inputs=|+-
  Sum3 : Sum  Inputs=|++-
  Sum4 : Sum  Inputs=|+++
  Sum5 : Sum  Inputs=|+-
  mdq0 : Outport
  wires:
  iqref/1 -> Sum5/1, Scope1/1
  Mux1/1 -> mdq0/1
  Sum4/1 -> [Eq], Mux1/2
  PID Controller1/1 -> Sum4/1
  Sum5/1 -> PID Controller1/1
  Constant4/1 -> Mux1/3
  Vd/1 -> Sum3/1
  Sum1/1 -> PID Controller/1
  iq/1 -> Sum5/2, Gain2/1, Scope1/2
  Vq/1 -> Sum4/2
  Gain1/1 -> Sum4/3
  id-ref/1 -> Sum1/1, Scope/1
  ipvd/1 -> Sum1/2, Gain1/1, Scope/2
  Gain2/1 -> Sum3/3
  Sum3/1 -> [Ed], Mux1/1
  PID Controller/1 -> Sum3/2

== system BESS_Harness/BESS/Detailed/BESS Controller/Grid Following/Reference Current ==
  note: Avoid division by zero during start
  note: Current Limiters
  V_ref : Inport
  V-mag : Inport  Port=2
  del f : Inport  Port=3
  LVRT_iq : Inport  Port=4
  PRef : Inport  Port=5
  QRef : Inport  Port=6
  Constant1 : Constant
  Constant3 : Constant  Value=Imax
  Current limits : Subsystem
  Refernce id generation : Subsystem
  Refernce iq generation : Subsystem
  Switch : Switch  Criteria=u2 ~= 0  SaturateOnIntegerOverflow=off  InputSameDT=off
  Unit Delay1 : UnitDelay  SampleTime=Ts
  Unit Delay3 : UnitDelay  SampleTime=Ts
  id_ref : Outport
  iq_ref : Outport  Port=2
  wires:
  Current limits/2(iubd) -> Refernce id generation/3(ubid)
  PRef/1 -> Refernce id generation/4(PRef)
  QRef/1 -> Refernce iq generation/5(Q_ref)
  Constant1/1 -> Switch/3
  Switch/1 -> Refernce iq generation/3(V_mag), Refernce id generation/1(V_mag)
  V-mag/1 -> Switch/2, Switch/1
  LVRT_iq/1 -> Refernce iq generation/4(LVRT_iq)
  Refernce iq generation/1(iq_ref) -> iq_ref/1, Unit Delay1/1
  V_ref/1 -> Refernce iq generation/2(V_ref)
  del f/1 -> Refernce id generation/2(del f)
  Refernce id generation/1(id_ref) -> Unit Delay3/1, id_ref/1
  Constant3/1 -> Current limits/1(Imax)
  Unit Delay3/1 -> Current limits/3(idref)
  Current limits/1(iubq) -> Refernce iq generation/1(ubiq)
  Unit Delay1/1 -> Current limits/2(iqref)

== system BESS_Harness/BESS/Detailed/BESS Controller/Grid Forming/Current Limiting ==
  In Bus Element : Inport  PortName=measure  Element=Igd
  In Bus Element1 : Inport  PortName=measure  Element=Igq
  In Bus Element2 : Inport  Port=2  PortName=reactiveControl  Element=Vmd
  In Bus Element4 : Inport  Port=2  PortName=reactiveControl  Element=Vmq
  CurrentLimitingMethod : Subsystem  Variant=on  VariantControlMode=label  VariantControl=Choice  LabelModeActiveChoice=ctSat
  Scope : Scope  NumInputPorts=2
  Subtract : Sum  Inputs=+-
  Subtract1 : Sum  Inputs=-+
  Out Bus Element : Outport  PortName=currentLimiting  Element=Vmd
  Out Bus Element1 : Outport  PortName=currentLimiting  Element=Vmq
  Out Bus Element2 : Outport  PortName=currentLimiting  Element=Idmax
  Out Bus Element3 : Outport  PortName=currentLimiting  Element=Iqmax
  wires:
  CurrentLimitingMethod/2(delVq) -> Subtract1/1
  CurrentLimitingMethod/1(delVd) -> Subtract/2
  CurrentLimitingMethod/3(Idmax) -> Out Bus Element2/1
  In Bus Element/1 -> CurrentLimitingMethod/1(Igd)  "Q"
  CurrentLimitingMethod/4(Iqmax) -> Out Bus Element3/1
  Subtract1/1 -> Out Bus Element1/1, Scope/2
  Subtract/1 -> Out Bus Element/1, Scope/1
  In Bus Element4/1 -> Subtract1/2
  In Bus Element1/1 -> CurrentLimitingMethod/2(Igq)
  In Bus Element2/1 -> Subtract/1

== system BESS_Harness/BESS/Detailed/BESS Controller/Grid Forming/Grid Voltage Reactive Power Support ==
  In Bus Element1 : Inport  PortName=measure  Element=Vgd
  In Bus Element3 : Inport  PortName=measure  Element=Vgq
  In Bus Element2 : Inport  PortName=measure  Element=Igd
  In Bus Element4 : Inport  PortName=measure  Element=Igq
  PrefInput : Inport  Port=2
  QrefInput : Inport  Port=3
  Modifying Active Power Reference : Subsystem
  Modifying Reactive Power Reference : Subsystem
  Scope : Scope
  Scope1 : Scope
      settings: ActiveDisplayYMinimum=0.9  ActiveDisplayYMaximum=1.1
  Scope2 : Scope
      settings: ActiveDisplayYMinimum=-1  ActiveDisplayYMaximum=1
  Pref : Outport
  Qref : Outport  Port=2
  wires:
  Modifying Reactive Power Reference/2(QrefNew) -> Qref/1, Scope2/1
  Modifying Reactive Power Reference/1(PrefNew) -> Pref/1, Scope1/1
  QrefInput/1 -> Modifying Reactive Power Reference/3(Qref)
  In Bus Element3/1 -> Modifying Reactive Power Reference/2(Vgq)
  In Bus Element1/1 -> Modifying Active Power Reference/2(Vd), Modifying Reactive Power Reference/1(Vgd)
  In Bus Element4/1 -> Modifying Active Power Reference/4(Igq)
  In Bus Element2/1 -> Modifying Active Power Reference/3(Igd)
  PrefInput/1 -> Modifying Active Power Reference/1(PrefInput)
  Modifying Active Power Reference/1(Pref) -> Modifying Reactive Power Reference/4(Pref), Scope/1

== system BESS_Harness/BESS/Detailed/BESS Controller/Grid Forming/Measurement ==
  Vgabcc : Inport
  Igabc : Inport  Port=2
  Angle : Inport  Port=3
  Frequency Measurement : Subsystem
  Gain1 : Gain  Gain=2/3
  Gain2 : Gain  Gain=2/3
  Gain3 : Gain  Gain=1%/(girdLineVoltage*sqrt(2/3))
  Gain4 : Gain  Gain=1%/(girdLineVoltage*sqrt(2/3))
  Gain5 : Gain  Gain=1%/(power/(sqrt(3)*girdLineVoltage)*sqrt(2))
  Gain6 : Gain  Gain=1%/(power/(sqrt(3)*girdLineVoltage)*sqrt(2))
  Power Measurement (Three-Phase) : eePowerMeasurement/Power Measurement (Three-Phase)  LabelModeActiveChoice=Discrete  F=powerFreq  K=[1]  Seq=Positive  Ts=measSampleTime
  abc2dq : Subsystem
  Out Bus Element : Outport  PortName=measure  Element=P
  Out Bus Element1 : Outport  PortName=measure  Element=Q
  Out Bus Element2 : Outport  PortName=measure  Element=Vgd
  Out Bus Element3 : Outport  PortName=measure  Element=Vgq
  Out Bus Element4 : Outport  PortName=measure  Element=Igd
  Out Bus Element5 : Outport  PortName=measure  Element=Igq
  Out Bus Element6 : Outport  PortName=measure  Element=fgrid
  Pmeas : Outport  Port=2
  Qmeas : Outport  Port=3
  fmeas : Outport  Port=4
  wires:
  Frequency Measurement/1(freq) -> fmeas/1, Out Bus Element6/1
  Gain6/1 -> Out Bus Element5/1  "Igq"
  Gain5/1 -> Out Bus Element4/1  "Igd"
  Gain4/1 -> Out Bus Element2/1  "Vgd"
  Gain3/1 -> Out Bus Element3/1  "Vgq"
  abc2dq/4(Igq) -> Gain6/1
  abc2dq/3(Igd) -> Gain5/1
  abc2dq/2(Vgq) -> Gain3/1
  abc2dq/1(Vgd) -> Gain4/1
  Gain1/1 -> Out Bus Element1/1, Qmeas/1  "Qmeas"
  Gain2/1 -> Out Bus Element/1, Pmeas/1  "Pmeas"
  Power Measurement (Three-Phase)/2 -> Gain1/1
  Igabc/1 -> Power Measurement (Three-Phase)/2, abc2dq/1(Igabc)  "Iabc"
  Power Measurement (Three-Phase)/1 -> Gain2/1
  Angle/1 -> abc2dq/2(Angle)
  Vgabcc/1 -> Power Measurement (Three-Phase)/1, Frequency Measurement/1(Vabc), abc2dq/3(Vgabc)  "Vabc"

== system BESS_Harness/BESS/Detailed/BESS Controller/Grid Forming/Power Control ==
  note: Active Power Control
  note: Reactive Power Control
  In Bus Element2 : Inport  PortName=measure  Element=P
  In Bus Element1 : Inport  PortName=measure  Element=fgrid
  BusElementIn : Inport  PortName=measure  Element=Vgd
  BusElementIn2 : Inport  PortName=measure  Element=Q
  Pref : Inport  Port=2
  Qref : Inport  Port=3
  Vref : Inport  Port=4
  Fref : Inport  Port=5
  CntrlFlag : Inport  Port=6
  ActivePowerControl : Subsystem  Variant=on  VariantControlMode=label  VariantControl=Choice  LabelModeActiveChoice=vsm
  ReactiveControl : Subsystem
  Scope : Scope
      settings: ActiveDisplayYMinimum=-13.20558  ActiveDisplayYMaximum=19.03908  DataLoggingVariableName=ScopeData16
  Out Bus Element : Outport  PortName=reactiveControl  Element=Vmd
  Out Bus Element1 : Outport  PortName=reactiveControl  Element=Vmq
  Out Bus Element6 : Outport  Port=2  PortName=activeControl  Element=angle
  Out Bus Element4 : Outport  Port=2  PortName=activeControl  Element=w
  angle : Outport  Port=3
  wires:
  BusElementIn2/1 -> ReactiveControl/3(Qmeas)
  BusElementIn/1 -> ReactiveControl/4(Vgdmeas), Scope/1
  [Cntrlflag] -> ReactiveControl/1(CntrlFlag)
  Vref/1 -> ReactiveControl/5(Vref)
  [Cntrlflag] -> ActivePowerControl/4(cntrlflag)
  CntrlFlag/1 -> [Cntrlflag]
  Fref/1 -> ActivePowerControl/3(fref)
  In Bus Element1/1 -> ActivePowerControl/5(fgrid)
  In Bus Element2/1 -> ActivePowerControl/2(Pmeas)
  Qref/1 -> ReactiveControl/2(Qref)  "Q"
  Pref/1 -> ActivePowerControl/1(Pref)  "Q"
  ReactiveControl/2(Vmq) -> Out Bus Element1/1
  ReactiveControl/1(Vmd) -> Out Bus Element/1
  ActivePowerControl/1(Theta) -> Out Bus Element6/1, angle/1
  ActivePowerControl/2(w) -> Out Bus Element4/1

== system BESS_Harness/BESS/Detailed/BESS Controller/Grid Forming/Subsystem2 ==
  In : Inport
  Reset : Inport  Port=2
  AND : Logic  IconShape=distinctive  AllPortsSameDT=off  OutDataTypeStr=boolean
  Data Type Conversion : DataTypeConversion  SaturateOnIntegerOverflow=off  RndMeth=Floor
  Delay : Delay  DelayLength=1  SampleTime=Ts*20000
  Delay1 : Delay  DelayLength=1
  NOT : Logic  Operator=NOT  IconShape=distinctive  AllPortsSameDT=off  OutDataTypeStr=boolean
  NOT1 : Logic  Operator=NOT  IconShape=distinctive  AllPortsSameDT=off  OutDataTypeStr=boolean
  Product : Product
  mabc : Outport
  wires:
  In/1 -> Product/2
  Reset/1 -> AND/1, Delay/1
  NOT/1 -> AND/2
  Delay/1 -> NOT/1
  Product/1 -> Delay1/1
  AND/1 -> NOT1/1
  NOT1/1 -> Data Type Conversion/1
  Data Type Conversion/1 -> Product/1
  Delay1/1 -> mabc/1

== system BESS_Harness/BESS/Detailed/BESS Controller/Grid Forming/VoltageCurrentControl ==
  In Bus Element : Inport  PortName=currentLimiting  Element=Vmd
  In Bus Element1 : Inport  PortName=currentLimiting  Element=Vmq
  In Bus Element6 : Inport  PortName=currentLimiting  Element=Idmax
  In Bus Element7 : Inport  PortName=currentLimiting  Element=Iqmax
  Bus Element In6 : Inport  Port=2  PortName=activeControl  Element=w
  Bus Element In1 : Inport  Port=2  PortName=activeControl  Element=angle
  Reset : Inport  Port=3
  In Bus Element2 : Inport  Port=4  PortName=measure  Element=Vgd
  In Bus Element3 : Inport  Port=4  PortName=measure  Element=Vgq
  In Bus Element4 : Inport  Port=4  PortName=measure  Element=Igd
  In Bus Element5 : Inport  Port=4  PortName=measure  Element=Igq
  Controller : Subsystem
      settings: PortSchema="{\"entries\":[{\"content\":{\"sides\":[{\"content\":{\"connectorIds\":[\"In1\",\"In2\",\"In3\",\"In4\",\"In5\",\"In6\",\"In7\",\"In8\",\"In9\"]},\"type\":\"ConnectorPlacement.EquallySpacedRectSide\",\"uuid\":\"29d30ab3-0ae0-4ae6-aaee-46c6f5faca9c\"},{\"content\":{\"connectorIds\":[\"Out1\",\"Out2\"],\"side\":\"RIGHT\"},\"type\":\"ConnectorPlacement.EquallySpacedRectSide\",\"uuid\":\"4918c3a7-9f8f-4af5-ac25-a0a0710917b2\"},{\"content\":{\"connectorIds\":[\"In10\"],\"side\":\"TOP\"},\"type\":\"ConnectorPlacement.EquallySpacedRectSide\",\"uuid\":\"c6ee8000-0a39-46c2-b8e8-8b73a56a82d9\"}]},\"type\":\"ConnectorPlacement.EquallySpacedConnector\",\"uuid\":\"193e0bc8-3764-41d1-9278-3938c4a9e9f5\"}],\"packageUris\":[\"http://schema.mathworks.com/mf0/Connector/R2020b\"],\"version\":\"1.0\"}"
  Modulation Signal : Subsystem
  mabc : Outport
  wires:
  Reset/1 -> Controller/10(Reset)
  Bus Element In1/1 -> Modulation Signal/3(Angle)
  In Bus Element1/1 -> Controller/3(Vgqref)
  In Bus Element/1 -> Controller/2(Vgdref)
  Bus Element In6/1 -> Controller/1(Angfreq)
  In Bus Element3/1 -> Controller/5(Vsq)
  In Bus Element2/1 -> Controller/4(Vsd)
  In Bus Element7/1 -> Controller/9(Iqmax)
  In Bus Element6/1 -> Controller/8(Idmax)
  In Bus Element5/1 -> Controller/7(Iq)
  In Bus Element4/1 -> Controller/6(Id)
  Controller/1(Vd) -> Modulation Signal/1(Vd)
  Modulation Signal/1(mabc) -> mabc/1
  Controller/2(Vq) -> Modulation Signal/2(Vq)

== system BESS_Harness/BESS/Detailed/BESS Plant/Converter/Average ==
  mabc : Inport
  Converter : ee_lib/Semiconductors & Converters/Converters/Average-Value Voltage Source Converter (Three-Phase)  port_option=ee.enum.threePhasePort.composite  frequency_option=ee.enum.converters.frequency.variable  input_option=ee.enum.converters.inputOption.ModWave  FRated=60 Hz  losses_parameterization=ee.enum.converters.losses.fixed  Pfixed=0.5 W  ks=0.01  kc1=1.7 V  kc2=0.01 Ohm  Ploss_vect=[100, 800, 1870, 3250, 4900] W  Irms_vect=[10, 100, 200, 300, 400] A  Vdc_nom=300 V  thermal_mass=30000 J/K  temperature_specify=off  temperature_priority=High  temperature=298.15 K  temperature_nominal_specify=off  temperature_nominal_value=1  temperature_nominal_unit=K
      settings: InternalSimscapePortConfiguration="{\"Bottom\":[],\"Left\":[{\"id\":\"ModWave\",\"label\":\"ModWave\",\"type\":\"input\"},{\"id\":\"N\",\"label\":\"~\",\"type\":\"foundation.electrical.three_phase\"}],\"Right\":[{\"id\":\"p\",\"label\":\"+\",\"type\":\"foundation.electrical.electrical\"},{\"id\":\"n\",\"label\":\"-\",\"type\":\"foundation.electrical.electrical\"}],\"Top\":[]}"
  Simulink-PS Converter : nesl_utility/Simulink-PS Converter  PhysicalDomain=network_engine_domain  SubClassName=ps_input  LeftPortType=input  RightPortType=output  PseudoPeriodic=off  Frequencies=[]  NoiseDistribution=none  NoiseParameters=[]  Unit=1  AffineConversion=off  FilteringAndDerivatives=provide  SimscapeFilterOrder=1  InputFilterTimeConstant=0.001  UdotUserProvided=0
  + : PMIOPort  Side=Left
  - : PMIOPort  Port=2  Side=Left
  ~ : PMIOPort  Port=3  Side=Right
  wires:
  mabc/1 -> Simulink-PS Converter/1
  connections:
  Simulink-PS Converter/RConn1 -- Converter/LConn1
  ~/RConn1 -- Converter/LConn2
  -/RConn1 -- Converter/RConn2
  +/RConn1 -- Converter/RConn1
